simulink library "lib_Convection_FCVertIncPlateCyl"  (R2015a)
settings: Solver=ode45  StartTime=0.0  StopTime=10.0  RelTol=1e-3
libraries: simulink x7
settings Model: Creator=jlkratz  LastModifiedBy=jlkratz

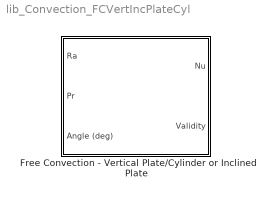
== system lib_Convection_FCVertIncPlateCyl ==
  Free Convection - Vertical Plate/Cylinder or Inclined Plate : Subsystem  mask(TSAT: Vertical Plate/Cylinder or Inclined Plate Free Convection){Corr_M=Correlation 2 - Laminar only (Ra < 10^9), PlateOrCyl_M=Plate, InclineOrVert_M=Inclined, DiamOverLen_M=1}
      mask prompts: Corr_M "Corr_M - Correlation"; DiamOverLen_M "DiamOverLen_M - Diameter to length ratio (cylinder only)"
      mask help:
      | This block estimates the average Nusselt number of free convecting flow over an isothermal vertical or inclined flat plate, or an isothermal vertical cylinder. For inclined vertical plates the correlation is only valid for the top surface of cold plates and bottom surface of hot plates. The bottom surface of cold plates and top surface of hot plates experience a complex 3-D flow that typically enhances heat transfer but is not able to be characterized by a generalized correlation. This block allows the user to select from 2 correlations which are described in the block help menu. Note that all fluid properrties should be evaluated at film temperature (average of the bulk fluid and surface temperatures). Note also that the Rayliegh number should be computed using the length of the plate or cylinder as the characteristic length.
      |
      | For more information see the help menu.
      mask init:
      | %setup inports -----------------------------------------------------------%
      | 
      | % Inport Numbers
      | n = 3; %first inport number
      | 
      | % Angle of plate (Angle)
      | if InclineOrVert_M == 2 && PlateOrCyl_M == 1
      |     if strcmp(get_param([gcb '/Angle (deg)'],'BlockType'),'Constant')
      |         MSK_ReplaceBlock_TMATS([gcb '/Angle (deg)'],'built-in/Inport');
      |     end
      |     set_param([gcb '/Angle (deg)'],'Port',num2str(n));
      |     n = n + 1;
      | else
      |     if strcmp(get_param([gcb '/Angle (deg)'],'BlockType'),'Inport')
      |         MSK_ReplaceBlock_TMATS([gcb '/Angle (deg)'],'built-in/Constant');
      |         set_param([gcb '/Angle (deg)'],'Value','0');
      |     end
      | end
      mask Help: web(which('Convection_TSAT_FCVertIncPlateCyl.html'),'-helpbrowser')
      mask TypeOptions Corr_M: Correlation 1 - Entire Ra range | Correlation 2 - Laminar only (Ra < 10^9)
      mask TypeOptions PlateOrCyl_M: Plate | Cylinder
      mask Callback PlateOrCyl_M:
      | sel = get_param(gcb,'PlateOrCyl_M');
      | if sel(1) == 'P'
      |     MSK_SEC_Enables3_TSAT('on',[3],'en')
      |     MSK_SEC_Enables3_TSAT('on',[4],'dis')
      | elseif sel(1) == 'C'
      |     MSK_SEC_Enables3_TSAT('on',[4],'en')
      |     MSK_SEC_Enables3_TSAT('on',[3],'dis')
      | end
      | clear sel
      mask TypeOptions InclineOrVert_M: Vertical | Inclined
      mask DialogControl Container13 Prompt: Plate Parameters
      mask DialogControl Container14 Prompt: Cylinder Parameters

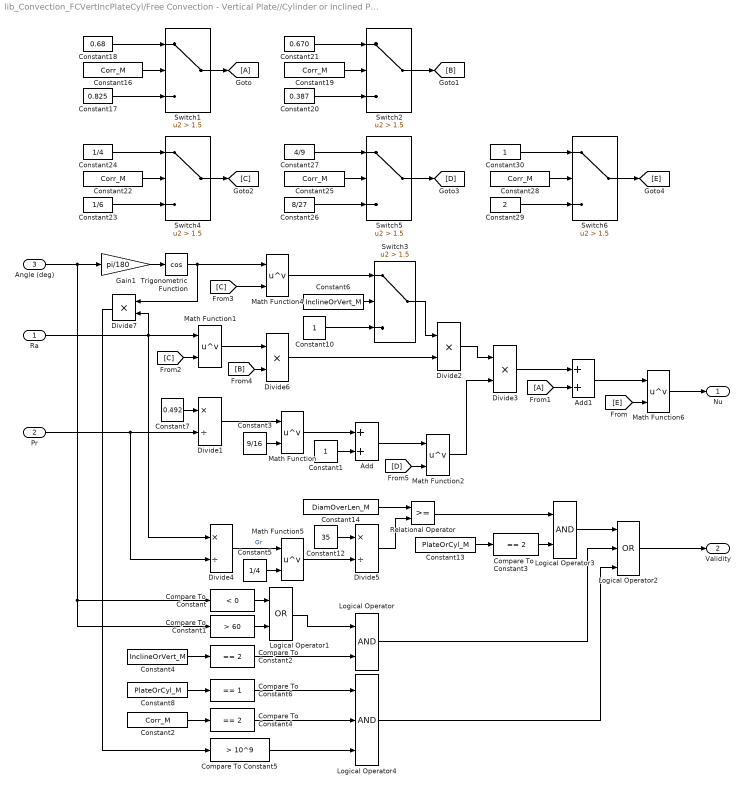
== system lib_Convection_FCVertIncPlateCyl/Free Convection - Vertical Plate//Cylinder or Inclined Plate ==
  Ra : Inport
  Pr : Inport  Port=2
  Angle (deg) : Inport  Port=3
  Add : Sum
  Add1 : Sum
  Compare To Constant : simulink/Logic and Bit Operations/Compare To Constant  relop=<  const=0  OutDataTypeStr=boolean
  Compare To Constant1 : simulink/Logic and Bit Operations/Compare To Constant  relop=>  const=60  OutDataTypeStr=boolean
  Compare To Constant2 : simulink/Logic and Bit Operations/Compare To Constant  relop===  const=2  OutDataTypeStr=boolean
  Compare To Constant3 : simulink/Logic and Bit Operations/Compare To Constant  relop===  const=2  OutDataTypeStr=boolean
  Compare To Constant4 : simulink/Logic and Bit Operations/Compare To Constant  relop===  const=2  OutDataTypeStr=boolean
  Compare To Constant5 : simulink/Logic and Bit Operations/Compare To Constant  relop=>  const=10^9  OutDataTypeStr=boolean
  Compare To Constant6 : simulink/Logic and Bit Operations/Compare To Constant  relop===  const=1  OutDataTypeStr=boolean
  Constant1 : Constant
  Constant10 : Constant
  Constant12 : Constant  Value=35
  Constant13 : Constant  Value=PlateOrCyl_M
  Constant14 : Constant  Value=DiamOverLen_M
  Constant{2,16,19,22,25,28} (6 alike) : Constant  Value=Corr_M
  Constant17 : Constant  Value=0.825
  Constant18 : Constant  Value=0.68
  Constant20 : Constant  Value=0.387
  Constant21 : Constant  Value=0.670
  Constant23 : Constant  Value=1/6
  Constant24 : Constant  Value=1/4
  Constant26 : Constant  Value=8/27
  Constant27 : Constant  Value=4/9
  Constant29 : Constant  Value=2
  Constant3 : Constant  Value=9/16
  Constant30 : Constant
  Constant4 : Constant  Value=InclineOrVert_M
  Constant5 : Constant  Value=1/4
  Constant6 : Constant  Value=InclineOrVert_M
  Constant7 : Constant  Value=0.492
  Constant8 : Constant  Value=PlateOrCyl_M
  Divide1 : Product  Inputs=*/
  Divide{2..3,6..7} (4 alike) : Product  Inputs=**
  Divide4 : Product  Inputs=*/
  Divide5 : Product  Inputs=*/
  Gain1 : Gain  Gain=pi/180
  Logical Operator : Logic  AllPortsSameDT=off  OutDataTypeStr=boolean
  Logical Operator1 : Logic  Operator=OR  AllPortsSameDT=off  OutDataTypeStr=boolean
  Logical Operator2 : Logic  Operator=OR  Inputs=3  AllPortsSameDT=off  OutDataTypeStr=boolean
  Logical Operator3 : Logic  AllPortsSameDT=off  OutDataTypeStr=boolean
  Logical Operator4 : Logic  Inputs=3  AllPortsSameDT=off  OutDataTypeStr=boolean
  Math Function{,1..2,4..6} (6 alike) : Math  Operator=pow  SaturateOnIntegerOverflow=on
  Relational Operator : RelationalOperator  OutDataTypeStr=boolean
  Switch{1..6} (6 alike) : Switch  Criteria=u2 > Threshold  Threshold=1.5
  Trigonometric Function : Trigonometry  Operator=cos
  Nu : Outport
  Validity : Outport  Port=2
  wires:
  Constant30/1 -> Switch6/1
  Constant29/1 -> Switch6/3
  Constant26/1 -> Switch5/3
  Constant27/1 -> Switch5/1
  Constant23/1 -> Switch4/3
  Constant24/1 -> Switch4/1
  Constant21/1 -> Switch2/1
  Constant20/1 -> Switch2/3
  Constant18/1 -> Switch1/1
  Constant17/1 -> Switch1/3
  Logical Operator4/1 -> Logical Operator2/3
  Compare To Constant5/1 -> Logical Operator4/3
  Compare To Constant4/1 -> Logical Operator4/2
  Compare To Constant6/1 -> Logical Operator4/1
  Constant8/1 -> Compare To Constant6/1
  Constant2/1 -> Compare To Constant4/1
  [E] -> Math Function6/2
  Switch6/1 -> [E]
  Constant28/1 -> Switch6/2
  Switch5/1 -> [D]
  Constant25/1 -> Switch5/2
  Switch4/1 -> [C]
  Constant22/1 -> Switch4/2
  Switch2/1 -> [B]
  Constant19/1 -> Switch2/2
  Switch1/1 -> [A]
  Constant16/1 -> Switch1/2
  [B] -> Divide6/2
  Logical Operator2/1 -> Validity/1
  Logical Operator/1 -> Logical Operator2/2
  Logical Operator3/1 -> Logical Operator2/1
  Compare To Constant3/1 -> Logical Operator3/2
  Relational Operator/1 -> Logical Operator3/1
  Divide5/1 -> Relational Operator/2
  Constant14/1 -> Relational Operator/1
  Constant13/1 -> Compare To Constant3/1
  Constant12/1 -> Divide5/1
  Math Function5/1 -> Divide5/2
  Constant5/1 -> Math Function5/2
  Logical Operator1/1 -> Logical Operator/1
  Compare To Constant1/1 -> Logical Operator1/2
  Compare To Constant/1 -> Logical Operator1/1
  Gain1/1 -> Trigonometric Function/1
  Compare To Constant2/1 -> Logical Operator/2
  Constant4/1 -> Compare To Constant2/1
  Divide4/1 -> Math Function5/1  "Gr"
  Switch3/1 -> Divide2/1
  Divide6/1 -> Divide2/2
  Divide2/1 -> Divide3/1
  Constant6/1 -> Switch3/2
  Math Function4/1 -> Switch3/1
  [C] -> Math Function4/2
  Trigonometric Function/1 -> Divide7/1, Math Function4/1
  Constant10/1 -> Switch3/3
  Math Function6/1 -> Nu/1
  Add1/1 -> Math Function6/1
  [A] -> Add1/2
  Divide3/1 -> Add1/1
  Math Function2/1 -> Divide3/2
  Add/1 -> Math Function2/1
  [D] -> Math Function2/2
  Math Function/1 -> Add/1
  Divide1/1 -> Math Function/1
  Pr/1 -> Divide4/2, Divide1/2
  Constant7/1 -> Divide1/1
  Constant3/1 -> Math Function/2
  Constant1/1 -> Add/2
  Math Function1/1 -> Divide6/1
  [C] -> Math Function1/2
  Ra/1 -> Divide7/2, Math Function1/1, Divide4/1
  Angle (deg)/1 -> Compare To Constant/1, Compare To Constant1/1, Gain1/1
  Divide7/1 -> Compare To Constant5/1
